simulink model "FW_formation_control"  (R2023b)
settings: Solver=ode45  StartTime=0.0  StopTime=80  RelTol=1e-3
values from neighbouring files (symbols this model uses):
  X8_lat_da_p_tf = X8_lat_p_tf(1)    [main.m]
  X8_lat_da_r_tf = X8_lat_r_tf(1)    [main.m]
  X8_lon_de_q_tf = X8_lon_q_tf(1)    [main.m]
  X8_lon_th_u_tf = X8_lon_u_tf(2)    [main.m]
  X8_lon_th_w_tf = X8_lon_w_tf(2)    [main.m]
undefined symbols (not defined in the file or in its folder): env, init, k_phi, k_theta, k_Va, X8
libraries: Fixed_Wing x1
settings Model: Creator=TigerWuu  LastModifiedBy=NCS
settings DebuggingCC: UnconnectedInputMsg=warning  UnconnectedOutputMsg=warning  UnconnectedLineMsg=warning
settings ModelReferenceCC: EnableRefExpFcnMdlSchedulingChecks=on
settings RTWCC: DLArmComputeVersion=19.05

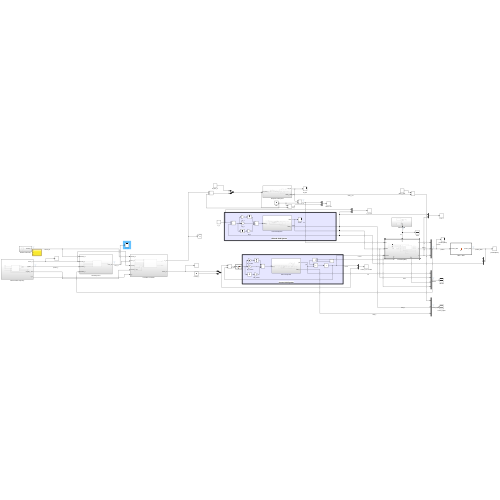
[thumbnail: Simulink's stored preview of the top-level diagram]
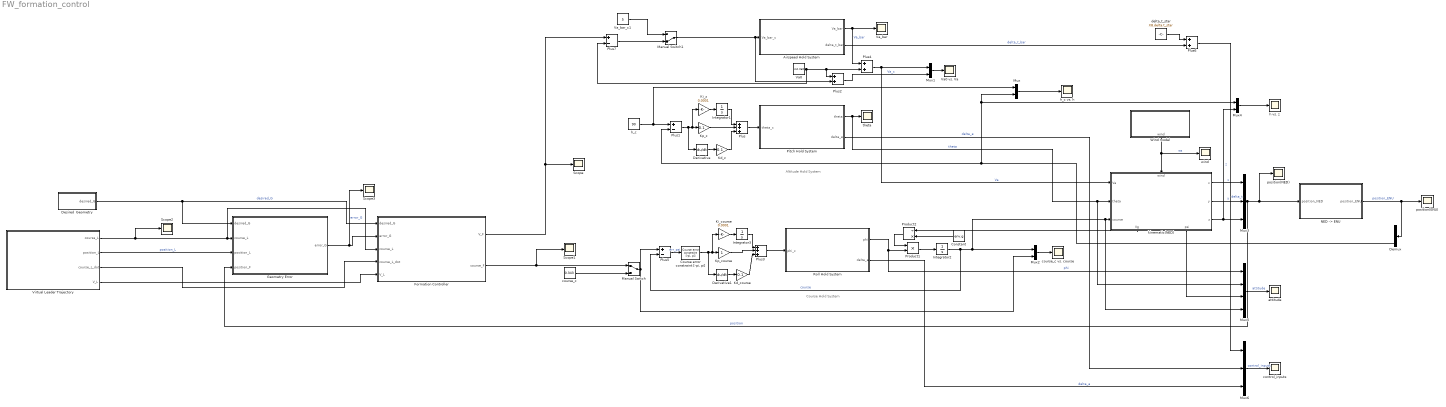
== system FW_formation_control ==
  note: Altitude Hold System
  note: Course Hold System
  Airspeed Hold System : Subsystem
  Constant : Constant  Value=env.g
  "Course error constraint [-pi, pi]" : Fixed_Wing/Fixed Wing Model/Course error constraint [-pi, pi]  SystemSampleTime=-1  VariantActivationTime=update diagram  AllowFlexibleInterface=on  Latency=0  AutoFrameSizeCalculation=off
      settings: SourceProductName=Fixed-Wing Model
  Demux : Demux  Outputs=3
  Derivative : Derivative
  Derivative1 : Derivative
  Desired  Geometry : Subsystem
  Formation Controller : Subsystem
  Geometry Error : Subsystem
  Integrator1 : Integrator
  Integrator2 : Integrator  InitialCondition=init.course0
  Integrator3 : Integrator
  Kd_course : Gain  Gain=0.1
  Kd_z : Gain  Gain=0.1
  Ki_course : Gain  Gain=0.0001
  Ki_z : Gain  Gain=0.0001
  Kp_course : Gain
  Kp_z : Gain  Gain=0.1
  Manual Switch : ManualSwitch
  Manual Switch1 : ManualSwitch  CurrentSetting=0
  Mux{,1..2,4} (4 alike) : Mux  Inputs=2
  Mux3 : Mux  Inputs=3
  Mux5 : Mux
  Mux6 : Mux  Inputs=3
  "NED -> ENU" : MATLAB Function  TreatAsAtomicUnit=on
  "Pitch Hold System " : Subsystem
      settings: ModelCloseFcn=function
  Plus : Sum  Inputs=+++
  Plus1 : Sum  Inputs=+-
  Plus2 : Sum
  Plus3 : Sum  Inputs=+++
  Plus4 : Sum
  Plus5 : Sum  Inputs=+-
  Plus6 : Sum
  Plus7 : Sum  Inputs=+-
  Product1 : Product
  Product2 : Product  Inputs=/*
  Roll Hold System : Subsystem
      settings: ModelCloseFcn=function
  Scope{,1..3} (4 alike) : Scope
  Va0 : Constant  Value=init.Va0
  Va0 vs. Va : Scope
  Va_bar : Scope
  Va_bar_c1 : Constant  Value=5
  Virtual Leader Trajectory : Subsystem
  Wind model : Subsystem
      settings: PortSchema="{\"entries\":[{\"content\":{\"sides\":[{\"content\":{},\"type\":\"ConnectorPlacement.EquallySpacedRectSide\",\"uuid\":\"19ef0eb7-c626-45ec-b76b-8668fc024824\"},{\"content\":{\"side\":\"RIGHT\"},\"type\":\"ConnectorPlacement.EquallySpacedRectSide\",\"uuid\":\"89e72569-ab94-4162-a6e2-b425ef08f724\"},{\"content\":{\"side\":\"TOP\"},\"type\":\"ConnectorPlacement.EquallySpacedRectSide\",\"uuid\":\"6d9409e9-6822-4cd9-902f-e5665cb68433\"},{\"content\":{\"connectorIds\":[\"Out1\"],\"side\":\"BOTTOM\"},\"type\":\"ConnectorPlacement.EquallySpacedRectSide\",\"uuid\":\"39a83352-0924-44fa-be5d-94a7c28bbbf3\"}]},\"type\":\"ConnectorPlacement.EquallySpacedConnector\",\"uuid\":\"6cf6ae00-ef23-42a2-99b2-ca60e191fb03\"}],\"packageUris\":[\"http://schema.mathworks.com/mf0/Connector/R2020b\"],\"version\":\"1.0\"}"
  attitude : Scope
  control_inputs : Scope
  course_c : Constant  Value=0.343
  course_c vs. course : Scope
  delta_t_star : Constant  Value=X8.delta.t_star
  h vs. z : Scope
  h_c : Constant  Value=90
  h_c vs. h : Scope
  kinematic(NED) : Subsystem
      settings: PortSchema="{\"entries\":[{\"content\":{\"sides\":[{\"content\":{\"connectorIds\":[\"In1\",\"In2\",\"In3\"]},\"type\":\"ConnectorPlacement.EquallySpacedRectSide\",\"uuid\":\"96d967d8-b822-4ab1-b08a-27adc20d5833\"},{\"content\":{\"connectorIds\":[\"Out1\",\"Out2\",\"Out3\"],\"side\":\"RIGHT\"},\"type\":\"ConnectorPlacement.EquallySpacedRectSide\",\"uuid\":\"505a36c9-cae2-422c-97bf-34d37872a31d\"},{\"content\":{\"connectorIds\":[\"In4\"],\"side\":\"TOP\"},\"type\":\"ConnectorPlacement.EquallySpacedRectSide\",\"uuid\":\"7bc53155-5df6-4b6a-9756-725497693b0a\"},{\"content\":{\"connectorIds\":[\"Out4\",\"Out5\"],\"side\":\"BOTTOM\"},\"type\":\"ConnectorPlacement.EquallySpacedRectSide\",\"uuid\":\"7777b465-a27e-4b61-9b89-f3b8fa4654d1\"}]},\"type\":\"ConnectorPlacement.EquallySpacedConnector\",\"uuid\":\"2150a812-5a4a-4a29-9c93-d226d95b2326\"}],\"packageUris\":[\"http://schema.mathworks.com/mf0/Connector/R2020b\"],\"version\":\"1.0\"}"
  position(ENU) : Scope
  position(NED) : Scope
  theta : Scope
  wind : Scope
  wires:
  "Pitch Hold System "/1(theta) -> kinematic(NED)/2(theta), Mux5/2, theta/1  "theta"
  Plus/1 -> "Pitch Hold System "/1(theta_c)
  Ki_z/1 -> Integrator1/1
  Integrator1/1 -> Plus/1
  Kp_z/1 -> Plus/2
  Plus1/1 -> Derivative/1, Ki_z/1, Kp_z/1
  h_c/1 -> Mux/1, Plus1/1
  Derivative/1 -> Kd_z/1
  Kd_z/1 -> Plus/3
  Manual Switch1/1 -> Plus2/2, Airspeed Hold System/1(Va_bar_c)
  Va0/1 -> Plus7/2, Plus2/1, Plus4/2
  Airspeed Hold System/1(Va_bar) -> Plus4/1, Va_bar/1  "Va_bar"
  Plus4/1 -> Mux1/1, kinematic(NED)/1(Va)  "Va"
  Mux/1 -> h_c vs. h/1
  Mux1/1 -> Va0 vs. Va/1
  Plus2/1 -> Mux1/2  "Va_c"
  Ki_course/1 -> Integrator3/1
  Mux2/1 -> course_c vs. course/1
  Roll Hold System/1(phi) -> Mux5/1, Product1/2  "phi"
  Manual Switch/1 -> Plus5/1, Mux2/2
  Product1/1 -> Integrator2/1
  Plus3/1 -> Roll Hold System/1(phi_c)
  Kd_course/1 -> Plus3/3
  Plus5/1 -> "Course error constraint [-pi, pi]"/1  "err_psi"
  Derivative1/1 -> Kd_course/1
  Kp_course/1 -> Plus3/2
  Integrator2/1 -> Mux5/4, kinematic(NED)/3(course), Mux2/1, Plus5/2  "course"
  Integrator3/1 -> Plus3/1
  Constant/1 -> Product2/2
  Product2/1 -> Product1/1
  kinematic(NED)/3(z) -> Mux4/2, Mux3/3  "z"
  kinematic(NED)/2(y) -> Mux3/2  "y"
  kinematic(NED)/1(x) -> Mux3/1  "x"
  Mux3/1 -> "NED -> ENU"/1(position_NED), position(NED)/1, Geometry Error/4(position_F)  "position"
  Mux4/1 -> h vs. z/1
  Mux5/1 -> attitude/1  "attitude"
  Airspeed Hold System/2(delta_t_bar) -> Plus6/2  "delta_t_bar"
  "Pitch Hold System "/2(delta_e) -> Mux6/2  "delta_e"
  Roll Hold System/2(delta_a) -> Mux6/3  "delta_a"
  Mux6/1 -> control_inputs/1  "control_inputs"
  delta_t_star/1 -> Plus6/1
  Plus6/1 -> Mux6/1  "delta_t"
  "NED -> ENU"/1(position_ENU) -> Demux/1, position(ENU)/1  "position_ENU"
  Wind model/1(wind) -> wind/1, kinematic(NED)/4(wind)  "ws"
  Demux/3 -> Mux/2, Mux4/1, Plus1/2
  kinematic(NED)/4(Vg) -> Product2/1
  kinematic(NED)/5(psi) -> Mux5/3
  Virtual Leader Trajectory/2(position_L) -> Geometry Error/3(position_L)  "position_L"
  Virtual Leader Trajectory/1(course_L) -> Scope2/1, Formation Controller/3(course_L), Geometry Error/2(course_L)
  Desired  Geometry/1(desired_G) -> Formation Controller/1(desired_G), Geometry Error/1(desired_G)  "desired_G"
  Virtual Leader Trajectory/3(course_L_dot) -> Formation Controller/4(course_L_dot)
  Virtual Leader Trajectory/4(V_L) -> Formation Controller/5(V_L)
  Geometry Error/1(error_G) -> Scope3/1, Formation Controller/2(error_G)  "error_G"
  course_c/1 -> Manual Switch/2
  Formation Controller/2(course_F) -> Scope1/1, Manual Switch/1
  Va_bar_c1/1 -> Manual Switch1/1
  Plus7/1 -> Manual Switch1/2
  Formation Controller/1(V_F) -> Plus7/1, Scope/1
  "Course error constraint [-pi, pi]"/1 -> Derivative1/1, Ki_course/1, Kp_course/1

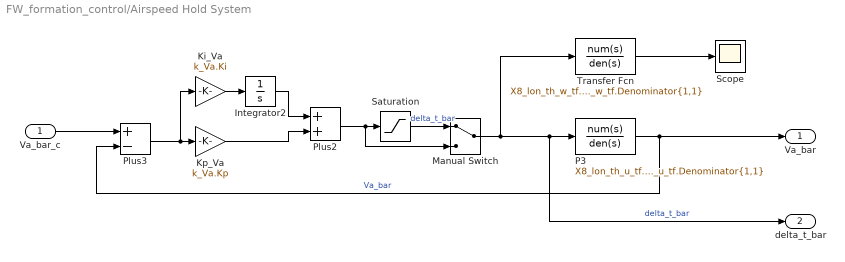
== system FW_formation_control/Airspeed Hold System ==
  Va_bar_c : Inport
  Integrator2 : Integrator
  Ki_Va : Gain  Gain=k_Va.Ki
  Kp_Va : Gain  Gain=k_Va.Kp
  Manual Switch : ManualSwitch
  P3 : TransferFcn  Numerator=X8_lon_th_u_tf.Numerator{1,1}  Denominator=X8_lon_th_u_tf.Denominator{1,1}
  Plus2 : Sum
  Plus3 : Sum  Inputs=+-
  Saturation : Saturate  UpperLimit=X8.delta.t_max-X8.delta.t_star  LowerLimit=X8.delta.t_min -X8.delta.t_star  LinearizeAsGain=off
  Scope : Scope
  Transfer Fcn : TransferFcn  Numerator=X8_lon_th_w_tf.Numerator{1,1}  Denominator=X8_lon_th_w_tf.Denominator{1,1}
  Va_bar : Outport
  delta_t_bar : Outport  Port=2
  wires:
  Ki_Va/1 -> Integrator2/1
  Plus3/1 -> Ki_Va/1, Kp_Va/1
  Va_bar_c/1 -> Plus3/1
  Kp_Va/1 -> Plus2/2
  Plus2/1 -> Manual Switch/2, Saturation/1
  Integrator2/1 -> Plus2/1
  P3/1 -> Va_bar/1, Plus3/2  "Va_bar"
  Manual Switch/1 -> Transfer Fcn/1, P3/1, delta_t_bar/1  "delta_t_bar"
  Transfer Fcn/1 -> Scope/1
  Saturation/1 -> Manual Switch/1  "delta_t_bar"

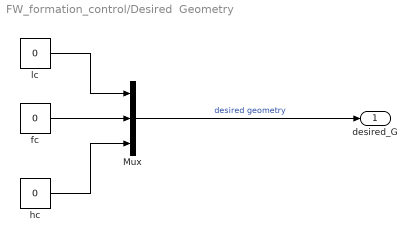
== system FW_formation_control/Desired  Geometry ==
  Mux : Mux  Inputs=3
  fc : Constant  Value=0
  hc : Constant  Value=0
  lc : Constant  Value=0
  desired_G : Outport
  wires:
  Mux/1 -> desired_G/1  "desired geometry"
  lc/1 -> Mux/1
  fc/1 -> Mux/2
  hc/1 -> Mux/3

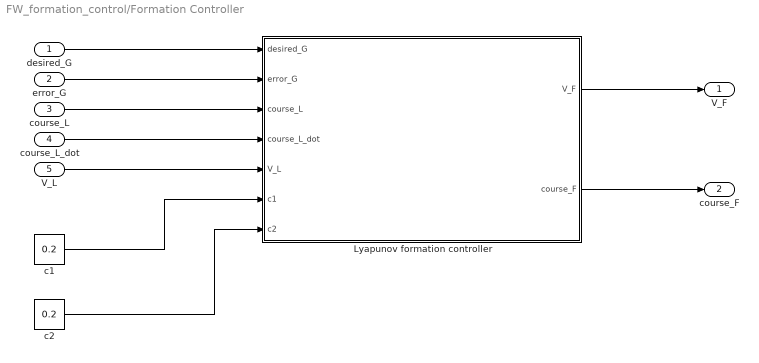
== system FW_formation_control/Formation Controller ==
  desired_G : Inport
  error_G : Inport  Port=2
  course_L : Inport  Port=3
  course_L_dot : Inport  Port=4
  V_L : Inport  Port=5
  Lyapunov formation controller : MATLAB Function  TreatAsAtomicUnit=on
  c1 : Constant  Value=0.2
  c2 : Constant  Value=0.2
  V_F : Outport
  course_F : Outport  Port=2
  wires:
  desired_G/1 -> Lyapunov formation controller/1(desired_G)
  error_G/1 -> Lyapunov formation controller/2(error_G)
  course_L/1 -> Lyapunov formation controller/3(course_L)
  course_L_dot/1 -> Lyapunov formation controller/4(course_L_dot)
  V_L/1 -> Lyapunov formation controller/5(V_L)
  c1/1 -> Lyapunov formation controller/6(c1)
  c2/1 -> Lyapunov formation controller/7(c2)
  Lyapunov formation controller/1(V_F) -> V_F/1
  Lyapunov formation controller/2(course_F) -> course_F/1

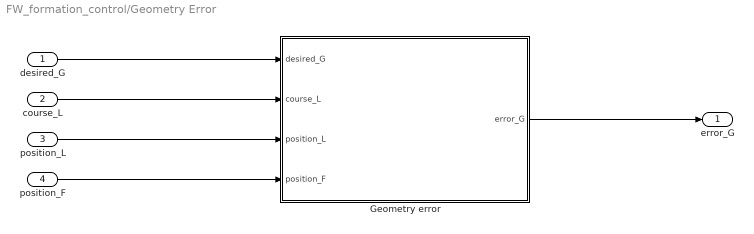
== system FW_formation_control/Geometry Error ==
  desired_G : Inport
  course_L : Inport  Port=2
  position_L : Inport  Port=3
  position_F : Inport  Port=4
  "Geometry error " : MATLAB Function  TreatAsAtomicUnit=on
  error_G : Outport
  wires:
  desired_G/1 -> "Geometry error "/1(desired_G)
  course_L/1 -> "Geometry error "/2(course_L)
  position_L/1 -> "Geometry error "/3(position_L)
  position_F/1 -> "Geometry error "/4(position_F)
  "Geometry error "/1(error_G) -> error_G/1

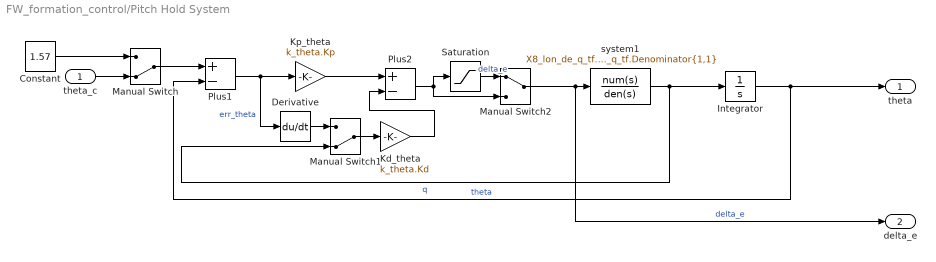
== system FW_formation_control/Pitch Hold System  ==
  theta_c : Inport
  Constant : Constant  Value=1.57
  Derivative : Derivative
  Integrator : Integrator  InitialCondition=init.theta0
  Kd_theta : Gain  Gain=k_theta.Kd
  Kp_theta : Gain  Gain=k_theta.Kp
  Manual Switch : ManualSwitch  CurrentSetting=0
  Manual Switch1 : ManualSwitch  CurrentSetting=0
  Manual Switch2 : ManualSwitch
  Plus1 : Sum  Inputs=+-
  Plus2 : Sum  Inputs=+-
  Saturation : Saturate  UpperLimit=X8.delta.e_max  LowerLimit=X8.delta.e_min
  system1 : TransferFcn  Numerator=X8_lon_de_q_tf.Numerator{1,1}  Denominator=X8_lon_de_q_tf.Denominator{1,1}
  theta : Outport
  delta_e : Outport  Port=2
  wires:
  system1/1 -> Manual Switch1/2, Integrator/1  "q"
  Plus2/1 -> Manual Switch2/2, Saturation/1
  Kp_theta/1 -> Plus2/1
  Plus1/1 -> Kp_theta/1, Derivative/1  "err_theta"
  Integrator/1 -> theta/1, Plus1/2  "theta"
  Constant/1 -> Manual Switch/1
  Manual Switch/1 -> Plus1/1
  theta_c/1 -> Manual Switch/2
  Manual Switch1/1 -> Kd_theta/1
  Derivative/1 -> Manual Switch1/1
  Kd_theta/1 -> Plus2/2
  Manual Switch2/1 -> delta_e/1, system1/1  "delta_e"
  Saturation/1 -> Manual Switch2/1  "delta_e"

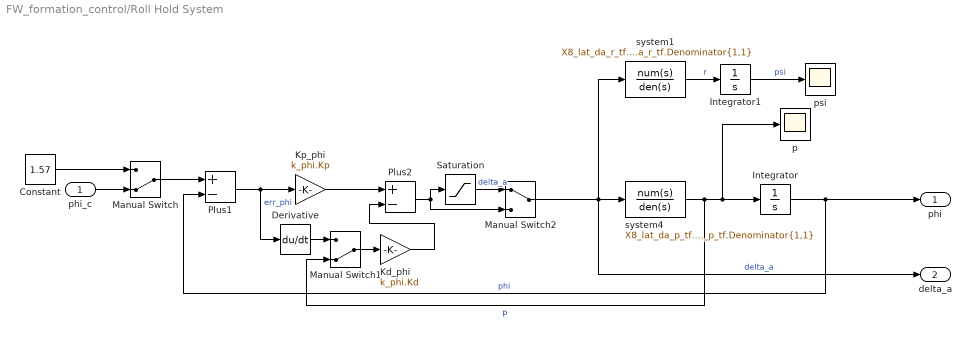
== system FW_formation_control/Roll Hold System ==
  phi_c : Inport
  Constant : Constant  Value=1.57
  Derivative : Derivative
  Integrator : Integrator  InitialCondition=init.phi0
  Integrator1 : Integrator  InitialCondition=init.psi0
  Kd_phi : Gain  Gain=k_phi.Kd
  Kp_phi : Gain  Gain=k_phi.Kp
  Manual Switch : ManualSwitch  CurrentSetting=0
  Manual Switch1 : ManualSwitch  CurrentSetting=0
  Manual Switch2 : ManualSwitch
  Plus1 : Sum  Inputs=+-
  Plus2 : Sum  Inputs=+-
  Saturation : Saturate  UpperLimit=X8.delta.a_max  LowerLimit=X8.delta.a_min  LinearizeAsGain=off
  p : Scope
  psi : Scope
  system1 : TransferFcn  Numerator=X8_lat_da_r_tf.Numerator{1,1}  Denominator=X8_lat_da_r_tf.Denominator{1,1}
  system4 : TransferFcn  Numerator=X8_lat_da_p_tf.Numerator{1,1}  Denominator=X8_lat_da_p_tf.Denominator{1,1}
  phi : Outport
  delta_a : Outport  Port=2
  wires:
  system4/1 -> Manual Switch1/2, p/1, Integrator/1  "p"
  Plus2/1 -> Manual Switch2/2, Saturation/1
  Kp_phi/1 -> Plus2/1
  Plus1/1 -> Kp_phi/1, Derivative/1  "err_phi"
  Integrator/1 -> phi/1, Plus1/2  "phi"
  Constant/1 -> Manual Switch/1
  Manual Switch/1 -> Plus1/1
  phi_c/1 -> Manual Switch/2
  Manual Switch1/1 -> Kd_phi/1
  Derivative/1 -> Manual Switch1/1
  Kd_phi/1 -> Plus2/2
  Manual Switch2/1 -> delta_a/1, system4/1, system1/1  "delta_a"
  system1/1 -> Integrator1/1  "r"
  Integrator1/1 -> psi/1  "psi"
  Saturation/1 -> Manual Switch2/1  "delta_a"

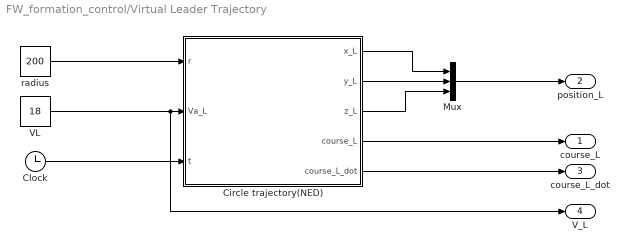
== system FW_formation_control/Virtual Leader Trajectory ==
  Circle trajectory(NED) : MATLAB Function  TreatAsAtomicUnit=on
  Clock : Clock
  Mux : Mux  Inputs=3
  VL : Constant  Value=18
  radius : Constant  Value=200
  course_L : Outport
  position_L : Outport  Port=2
  course_L_dot : Outport  Port=3
  V_L : Outport  Port=4
  wires:
  radius/1 -> Circle trajectory(NED)/1(r)
  VL/1 -> V_L/1, Circle trajectory(NED)/2(Va_L)
  Clock/1 -> Circle trajectory(NED)/3(t)
  Mux/1 -> position_L/1
  Circle trajectory(NED)/1(x_L) -> Mux/1
  Circle trajectory(NED)/2(y_L) -> Mux/2
  Circle trajectory(NED)/5(course_L_dot) -> course_L_dot/1
  Circle trajectory(NED)/4(course_L) -> course_L/1
  Circle trajectory(NED)/3(z_L) -> Mux/3

== system FW_formation_control/Wind model ==
  Manual Switch : ManualSwitch  CurrentSetting=0
  "Steady Wind " : Subsystem
  no wind : Subsystem
  wind : Outport
  wires:
  "Steady Wind "/1(ws) -> Manual Switch/1
  no wind/1(wind) -> Manual Switch/2
  Manual Switch/1 -> wind/1  "ws"

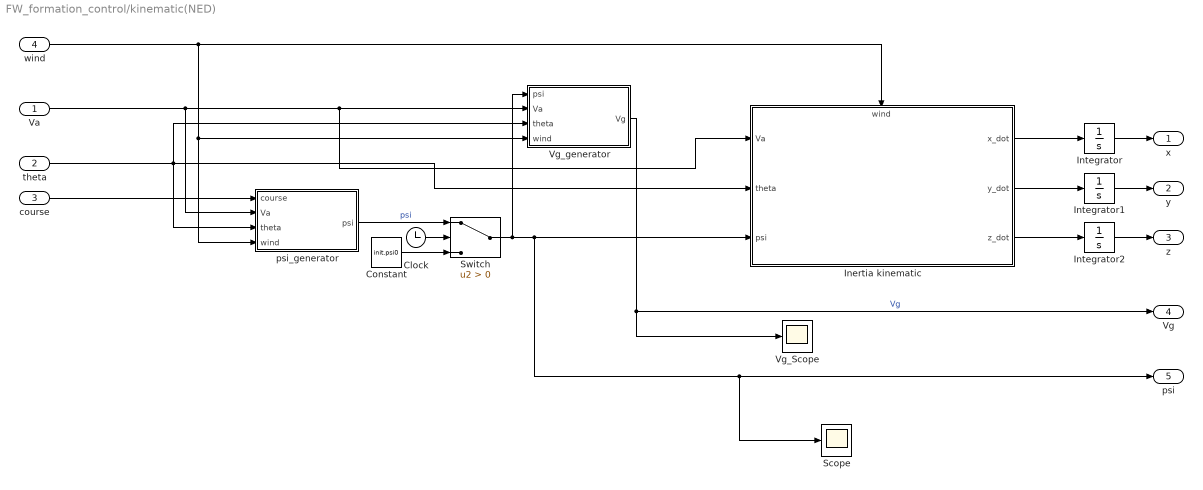
== system FW_formation_control/kinematic(NED) ==
  Va : Inport
  theta : Inport  Port=2
  course : Inport  Port=3
  wind : Inport  Port=4
  Clock : Clock
  Constant : Constant  Value=init.psi0
  Inertia kinematic : Subsystem
      settings: PortSchema="{\"entries\":[{\"content\":{\"sides\":[{\"content\":{\"connectorIds\":[\"In1\",\"In2\",\"In3\"]},\"type\":\"ConnectorPlacement.EquallySpacedRectSide\",\"uuid\":\"18991cbd-8d8f-4668-8054-d56b6b4d2674\"},{\"content\":{\"connectorIds\":[\"Out1\",\"Out2\",\"Out3\"],\"side\":\"RIGHT\"},\"type\":\"ConnectorPlacement.EquallySpacedRectSide\",\"uuid\":\"98d568d4-17ea-4287-b7bc-cb3e53942fc3\"},{\"content\":{\"connectorIds\":[\"In4\"],\"side\":\"TOP\"},\"type\":\"ConnectorPlacement.EquallySpacedRectSide\",\"uuid\":\"972ca0ea-c255-483c-a17b-ab0326bdc39e\"}]},\"type\":\"ConnectorPlacement.EquallySpacedConnector\",\"uuid\":\"0db01b3b-f146-4ef8-8588-0b44af2f41d6\"}],\"packageUris\":[\"http://schema.mathworks.com/mf0/Connector/R2020b\"],\"version\":\"1.0\"}"
  Integrator : Integrator  InitialCondition=init.x0
  Integrator1 : Integrator  InitialCondition=init.y0
  Integrator2 : Integrator  InitialCondition=init.z0
  Scope : Scope
  Switch : Switch  Criteria=u2 > Threshold  SaturateOnIntegerOverflow=off  InputSameDT=off
  Vg_Scope : Scope
  Vg_generator : MATLAB Function  TreatAsAtomicUnit=on
  "psi_generator " : MATLAB Function  TreatAsAtomicUnit=on
  x : Outport
  y : Outport  Port=2
  z : Outport  Port=3
  Vg : Outport  Port=4
  psi : Outport  Port=5
  wires:
  Integrator2/1 -> z/1
  Integrator/1 -> x/1
  Integrator1/1 -> y/1
  Va/1 -> Vg_generator/2(Va), Inertia kinematic/1(Va), "psi_generator "/2(Va)
  course/1 -> "psi_generator "/1(course)
  theta/1 -> Inertia kinematic/2(theta), Vg_generator/3(theta), "psi_generator "/3(theta)
  wind/1 -> Inertia kinematic/4(wind), Vg_generator/4(wind), "psi_generator "/4(wind)
  Vg_generator/1(Vg) -> Vg_Scope/1, Vg/1  "Vg"
  Inertia kinematic/1(x_dot) -> Integrator/1
  Inertia kinematic/2(y_dot) -> Integrator1/1
  Inertia kinematic/3(z_dot) -> Integrator2/1
  Switch/1 -> Vg_generator/1(psi), Inertia kinematic/3(psi), Scope/1, psi/1
  Clock/1 -> Switch/2
  "psi_generator "/1(psi) -> Switch/1  "psi"
  Constant/1 -> Switch/3

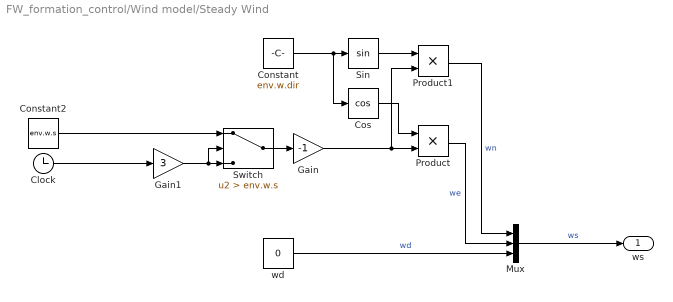
== system FW_formation_control/Wind model/Steady Wind  ==
  Clock : Clock
  Constant : Constant  Value=env.w.dir
  Constant2 : Constant  Value=env.w.s
  Cos : Trigonometry  Operator=cos
  Gain : Gain  Gain=-1
  Gain1 : Gain  Gain=3
  Mux : Mux  Inputs=3
  Product : Product
  Product1 : Product
  Sin : Trigonometry
  Switch : Switch  Criteria=u2 > Threshold  Threshold=env.w.s  SaturateOnIntegerOverflow=off  InputSameDT=off
  wd : Constant  Value=0
  ws : Outport
  wires:
  wd/1 -> Mux/3  "wd"
  Mux/1 -> ws/1  "ws"
  Product1/1 -> Mux/1  "wn"
  Product/1 -> Mux/2  "we"
  Constant/1 -> Cos/1, Sin/1
  Cos/1 -> Product/1
  Sin/1 -> Product1/1
  Gain/1 -> Product1/2, Product/2
  Clock/1 -> Gain1/1
  Gain1/1 -> Switch/2, Switch/3
  Constant2/1 -> Switch/1
  Switch/1 -> Gain/1

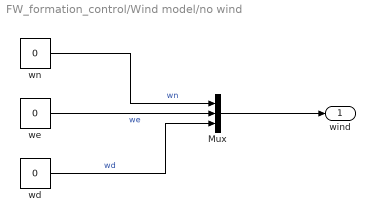
== system FW_formation_control/Wind model/no wind ==
  Mux : Mux  Inputs=3
  wd : Constant  Value=0
  we : Constant  Value=0
  wn : Constant  Value=0
  wind : Outport
  wires:
  wd/1 -> Mux/3  "wd"
  Mux/1 -> wind/1
  wn/1 -> Mux/1  "wn"
  we/1 -> Mux/2  "we"

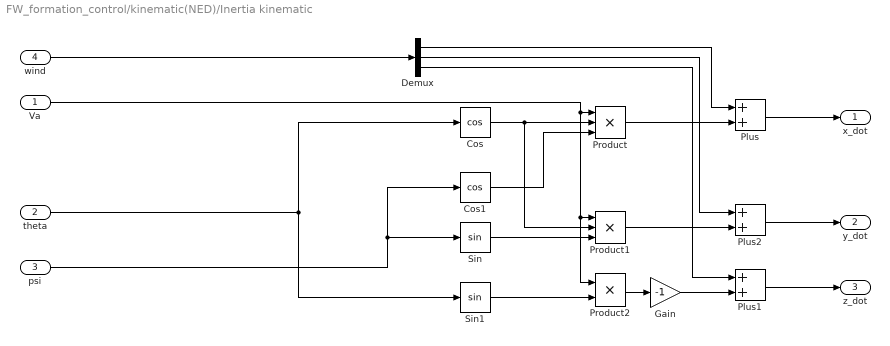
== system FW_formation_control/kinematic(NED)/Inertia kinematic ==
  Va : Inport
  theta : Inport  Port=2
  psi : Inport  Port=3
  wind : Inport  Port=4
  Cos : Trigonometry  Operator=cos
  Cos1 : Trigonometry  Operator=cos
  Demux : Demux  Outputs=3
  Gain : Gain  Gain=-1
  Plus : Sum
  Plus1 : Sum
  Plus2 : Sum
  Product : Product  Inputs=3
  Product1 : Product  Inputs=3
  Product2 : Product
  Sin : Trigonometry
  Sin1 : Trigonometry
  x_dot : Outport
  y_dot : Outport  Port=2
  z_dot : Outport  Port=3
  wires:
  Va/1 -> Product2/1, Product1/1, Product/1
  Demux/3 -> Plus1/1
  Demux/2 -> Plus2/1
  Demux/1 -> Plus/1
  Plus/1 -> x_dot/1
  Plus2/1 -> y_dot/1
  Product/1 -> Plus/2
  Product1/1 -> Plus2/2
  Plus1/1 -> z_dot/1
  Sin1/1 -> Product2/2
  Cos/1 -> Product/2, Product1/2
  Product2/1 -> Gain/1
  Gain/1 -> Plus1/2
  Sin/1 -> Product1/3
  Cos1/1 -> Product/3
  theta/1 -> Cos/1, Sin1/1
  psi/1 -> Cos1/1, Sin/1
  wind/1 -> Demux/1

== matlab function FW_formation_control/kinematic(NED)/psi_generator  ==
  data: course input; psi output; Va input; theta input; wind input
function psi = fcn(course, Va, theta, wind)
    psi = course-asin(1/(Va*cos(theta))*wind(1:2)'*[-sin(course);cos(course)]);
end

== matlab function FW_formation_control/NED -> ENU ==
  data: position_NED input; position_ENU output
function position_ENU = fcn(position_NED)
R_NED_ENU = [0 1 0;
             1 0 0;
             0 0 -1;];
position_ENU = R_NED_ENU* position_NED;
end

== matlab function FW_formation_control/kinematic(NED)/Vg_generator ==
  data: psi input; Vg output; Va input; theta input; wind input
function Vg = fcn(psi, Va, theta, wind)
    Vw = norm(wind);
    Vg = sqrt(Va^2+Vw^2+2*Va*[cos(psi)*cos(theta);sin(psi)*cos(theta);-sin(theta)]'*wind);
end

== matlab function FW_formation_control/Virtual Leader Trajectory/Circle trajectory(NED) ==
  data: x_L output; y_L output; z_L output; course_L output; course_L_dot output; r input; Va_L input; t input
function [x_L, y_L, z_L, course_L,course_L_dot] = trajectory_generation(r,Va_L, t)
    omega = Va_L/r; % rad/s
    y_L = r*cos(omega*t);
    x_L = r*sin(omega*t);
    z_L = -90;
    y_L_dot = -r*omega*sin(omega*t);
    x_L_dot = r*omega*cos(omega*t);
    y_L_dotdot = -r*omega^2*cos(omega*t);
    x_L_dotdot = -r*omega^2*sin(omega*t);
    course_L = atan2(y_L_dot,x_L_dot);
    course_L_dot = (y_L_dotdot*x_L_dot-x_L_dotdot*y_L_dot)/(x_L_dot^2+y_L_dot^2);
end

== matlab function FW_formation_control/Geometry Error/Geometry error  ==
  data: desired_G input; course_L input; error_G output; position_L input; position_F input
function error_G = geometry_error_generation(desired_G, course_L, position_L, position_F)
    error_G = [sin(course_L), -cos(course_L) ; cos(course_L), sin(course_L)]*[position_L(1) - position_F(1); position_L(2)-position_F(2)] - [desired_G(1) ; desired_G(2)];
    % error_G = [error_G ; position_L(3)-position_F(3)-desired_G(3)];

end

== matlab function FW_formation_control/Formation Controller/Lyapunov formation controller ==
  data: desired_G input; V_F output; error_G input; course_L input; course_L_dot input; V_L input; c1 input; c2 input; course_F output
function [V_F, course_F] = lyapunov_formation(desired_G, error_G, course_L, course_L_dot, V_L,  c1, c2)
    lc = desired_G(1);
    fc = desired_G(2);
    le = error_G(1);
    fe = error_G(2);
    V_F = sqrt((c1*le+course_L_dot*(fe+fc))^2+(c2*fe-course_L_dot*(le+lc)+V_L)^2);
    course_F = atan2(-c1*le-course_L_dot*(fe+fc), c2*fe-course_L_dot*(le+lc)+V_L)+course_L;
end
